simulink model "Commande_a_R2015a"  (R2015a)
settings: Solver=ode45  SolverMode=SingleTasking  StartTime=0.0  StopTime=10  RelTol=1e-3
settings Model: CovMetricSettings=dwe  CovHtmlReporting=off  covSaveCumulativeToWorkspaceVar=off  CovSaveSingleToWorkspaceVar=off  CovExternalEMLEnable=on  Creator=USER  LastModifiedBy=USER
settings DataIOCC: LimitDataPoints=off  SaveFormat=Dataset
settings DebuggingCC: SFUnexpectedBacktrackingDiag=error  SFNoUnconditionalDefaultTransitionDiag=error
settings HardwareCC: ProdBitPerPointer=64  ProdLargestAtomicFloat=Float  ProdIntDivRoundTo=Zero  ProdEndianess=LittleEndian  ProdHWDeviceType=Specified
settings ModelReferenceCC: PropagateSignalLabelsOutOfModel=on
settings SFSimCC: SimUseLocalCustomCode=on
settings RTWCC: RTWUseLocalCustomCode=on
settings GRTTargetCC: TargetLangStandard=C99 (ISO)  GeneratePreprocessorConditionals=Use local settings

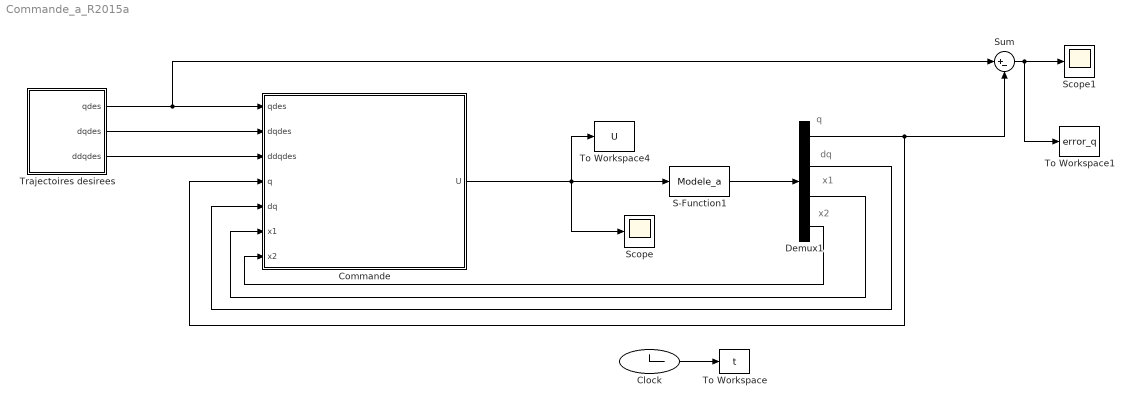
== system Commande_a_R2015a ==
  note: q
  note: dq
  note: x1
  note: x2
  Clock : Clock
  Commande : Subsystem
  Demux1 : Demux
  S-Function1 : S-Function  FunctionName=Modele_a  SFunctionDeploymentMode=off  EnableBusSupport=off
  Scope : Scope
      settings: TimeRange=auto  MaxDataPoints=5000  SaveToWorkspace=off  SaveName=ScopeData  YMin=-3881.13142  YMax=8575.16183  SampleTime=-1
  Scope1 : Scope
      settings: TimeRange=auto  MaxDataPoints=5000  SaveToWorkspace=off  YMin=-0.00044  YMax=0.00127  SampleTime=-1
  Sum : Sum  Inputs=|+-
  To Workspace : ToWorkspace  VariableName=t  SampleTime=-1
  To Workspace1 : ToWorkspace  VariableName=error_q  SampleTime=-1
  To Workspace4 : ToWorkspace  VariableName=U  SampleTime=-1
  Trajectoires desirees : Subsystem
  wires:
  Commande/1(U) -> To Workspace4/1, S-Function1/1, Scope/1
  S-Function1/1 -> Demux1/1
  Demux1/2 -> Commande/5(dq)
  Demux1/3 -> Commande/6(x1)
  Demux1/4 -> Commande/7(x2)
  Trajectoires desirees/1(qdes) -> Sum/1, Commande/1(qdes)
  Trajectoires desirees/2(dqdes) -> Commande/2(dqdes)
  Trajectoires desirees/3(ddqdes) -> Commande/3(ddqdes)
  Demux1/1 -> Sum/2, Commande/4(q)
  Sum/1 -> To Workspace1/1, Scope1/1
  Clock/1 -> To Workspace/1

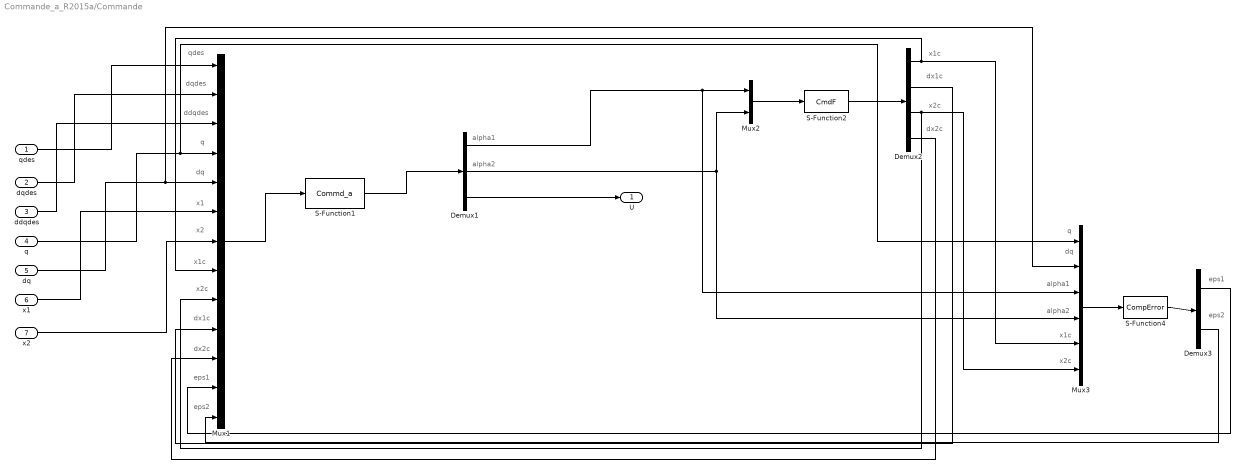
== system Commande_a_R2015a/Commande ==
  note: q
  note: dq
  note: alpha1
  note: alpha2
  note: x1c
  note: x2c
  note: eps1
  note: eps2
  note: x1c
  note: dx1c
  note: x2c
  note: dx2c
  note: alpha1
  note: alpha2
  note: qdes
  note: dqdes
  note: ddqdes
  note: q
  note: dq
  note: x1
  note: x2
  note: x1c
  note: x2c
  note: dx1c
  note: dx2c
  note: eps1
  note: eps2
  qdes : Inport
  dqdes : Inport  Port=2
  ddqdes : Inport  Port=3
  q : Inport  Port=4
  dq : Inport  Port=5
  x1 : Inport  Port=6
  x2 : Inport  Port=7
  Demux1 : Demux  Outputs=3
  Demux2 : Demux
  Demux3 : Demux  Outputs=2
  Mux1 : Mux  Inputs=13
  Mux2 : Mux  Inputs=2
  Mux3 : Mux  Inputs=6
  S-Function1 : S-Function  FunctionName=Commd_a  SFunctionDeploymentMode=off  EnableBusSupport=off
  S-Function2 : S-Function  FunctionName=CmdF  SFunctionDeploymentMode=off  EnableBusSupport=off
  S-Function4 : S-Function  FunctionName=CompError  SFunctionDeploymentMode=off  EnableBusSupport=off
  U : Outport
  wires:
  Mux2/1 -> S-Function2/1
  Mux1/1 -> S-Function1/1
  S-Function1/1 -> Demux1/1
  S-Function2/1 -> Demux2/1
  Demux1/3 -> U/1
  Mux3/1 -> S-Function4/1
  S-Function4/1 -> Demux3/1
  Demux1/1 -> Mux3/3, Mux2/1
  Demux1/2 -> Mux2/2, Mux3/4
  qdes/1 -> Mux1/1
  dqdes/1 -> Mux1/2
  ddqdes/1 -> Mux1/3
  q/1 -> Mux1/4, Mux3/1
  dq/1 -> Mux1/5, Mux3/2
  x1/1 -> Mux1/6
  x2/1 -> Mux1/7
  Demux3/2 -> Mux1/13
  Demux3/1 -> Mux1/12
  Demux2/1 -> Mux1/8, Mux3/5
  Demux2/3 -> Mux1/9, Mux3/6
  Demux2/2 -> Mux1/10
  Demux2/4 -> Mux1/11

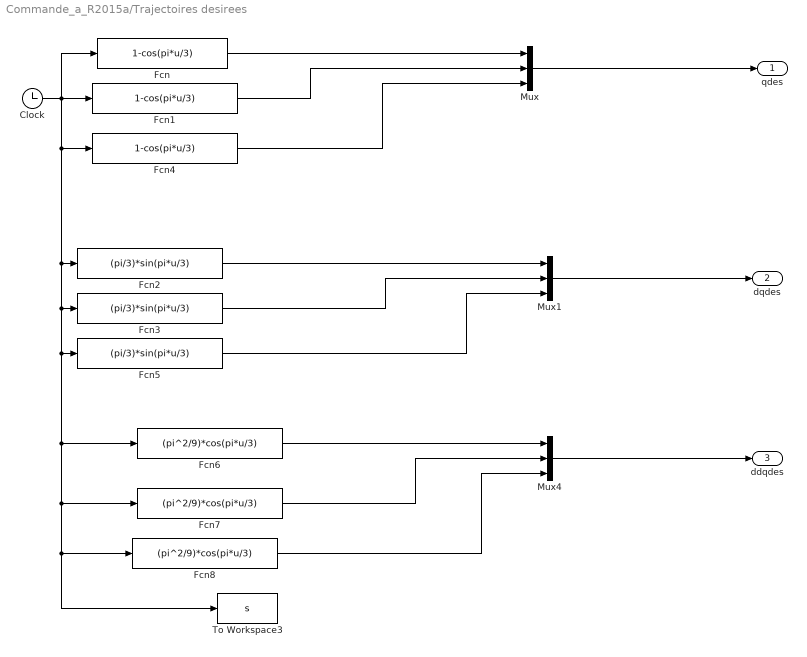
== system Commande_a_R2015a/Trajectoires desirees ==
  Clock : Clock
  Fcn : Fcn  Expr=1-cos(pi*u/3)
  Fcn1 : Fcn  Expr=1-cos(pi*u/3)
  Fcn2 : Fcn  Expr=(pi/3)*sin(pi*u/3)
  Fcn3 : Fcn  Expr=(pi/3)*sin(pi*u/3)
  Fcn4 : Fcn  Expr=1-cos(pi*u/3)
  Fcn5 : Fcn  Expr=(pi/3)*sin(pi*u/3)
  Fcn6 : Fcn  Expr=(pi^2/9)*cos(pi*u/3)
  Fcn7 : Fcn  Expr=(pi^2/9)*cos(pi*u/3)
  Fcn8 : Fcn  Expr=(pi^2/9)*cos(pi*u/3)
  Mux : Mux  Inputs=3
  Mux1 : Mux  Inputs=3
  Mux4 : Mux  Inputs=3
  To Workspace3 : ToWorkspace  VariableName=s  SampleTime=-1
  qdes : Outport
  dqdes : Outport  Port=2
  ddqdes : Outport  Port=3
  wires:
  Mux1/1 -> dqdes/1
  Mux/1 -> qdes/1
  Mux4/1 -> ddqdes/1
  Fcn/1 -> Mux/1
  Fcn4/1 -> Mux/3
  Fcn1/1 -> Mux/2
  Fcn2/1 -> Mux1/1
  Fcn3/1 -> Mux1/2
  Fcn5/1 -> Mux1/3
  Clock/1 -> Fcn6/1, Fcn7/1, To Workspace3/1, Fcn8/1, Fcn5/1, Fcn3/1, Fcn2/1, Fcn4/1, Fcn/1, Fcn1/1
  Fcn6/1 -> Mux4/1
  Fcn7/1 -> Mux4/2
  Fcn8/1 -> Mux4/3
